simulink library "qrd_matrix_library"  (Simulink 8.7)
settings: Solver=ode45  StartTime=0.0  StopTime=10.0  RelTol=1e-3
values from neighbouring files (symbols this model uses):
  vectorization = 2    [qrd_test.m]
undefined symbols (not defined in the file or in its folder): AdvDSPBChannelOutDisplay, AdvDSPBDMemDisplay, Back_Substitution_instances, column_count, column_count_1, column_count_2, dpoly, dspba_ChannelInVis, dspba_ChannelOutVis, dspba_internal_get_channel_ports, evalAionMaskParam, latency, primtype, QRD_vectorization, recipsqrt, row, row_count, row_count_1, row_count_2, UseDontCare, value, x
libraries: DSPBAPrim x683, DSPBAControl x37, qrd_matrix_library x33, DSPBAVectorUtil x6, DSPBAVectorPrim x3
(part 6 of 8)

== system qrd_matrix_library/QR_decomposition/Data Mux ==
  Valid In : Inport
  Channel In : Inport  Port=2
  r2_k_k_valid_in : Inport  Port=3
  rn_k_j_valid_in : Inport  Port=4
  A_j_update_valid_in : Inport  Port=5
  Q_k_valid_in : Inport  Port=6
  Input_Memory_Read_Data : Inport  Port=7
  A_k_Memory_Read_Data : Inport  Port=8
  rn_k_j_over_r2_k_k_fifo_Data : Inport  Port=9
  inv_r_k_k_Data : Inport  Port=10
  Dot_Product_Acc_Init_In : Inport  Port=11
  r2_k_k_Acc_Valid_In : Inport  Port=12
  rn_k_j_Acc_Valid_In : Inport  Port=13
  A_j_Address_In : Inport  Port=14
  A_j_Update_last_Valid_In : Inport  Port=15
  Done_In : Inport  Port=16
  ChannelIn : DSPBAPrim/ChannelIn  primtype=channelin  nInputs=dspba_internal_get_channel_ports(gcb)  nOutputs=dspba_internal_get_channel_ports(gcb)  omode=Inherit via internal rule  otype=sfix(16)  scale=2^-15  rndmethod=Unbiased  factor=1  satmethod=Symmetric  shift_vec=[0 1 2 -1]  value=14  inPortNames=['v'; 'c'; '0'; '1'; '2'; '3'; '4'; '5'; '6'; '7'; '8'; '9'; 'A'; 'B'; 'D'; 'E'; 'F'; 'G'; 'H'; 'I'; 'J'; 'K'; 'L'; 'M'; 'N'; 'O'; 'P'; 'Q'; 'R'; 'S'; 'T'; 'U'; 'W'; 'X'; 'Y'; 'Z']  outPortNames=['v'; 'c'; '0'; '1'; '2'; '3'; '4'; '5'; '6'; '7'; '8'; '9'; 'A'; 'B'; 'D'; 'E'; 'F'; 'G'; 'H'; 'I'; 'J'; 'K'; 'L'; 'M'; 'N'; 'O'; 'P'; 'Q'; 'R'; 'S'; 'T'; 'U'; 'W'; 'X'; 'Y'; 'Z']  dspbaimage=dspba_prim.jpg  text=fprintf('In');  style=Optimised  dataSignals=14  foldingEnabled=off  channels=1  sampleRate=200  packetBeginPresent=off  packetBeginEnabled=off  visibilities=dspba_ChannelInVis(gcb)  latencyCorrection=0  version=20141013
  ChannelOut : DSPBAPrim/ChannelOut  primtype=channelout  nInputs=dspba_internal_get_channel_ports(gcb)  nOutputs=dspba_internal_get_channel_ports(gcb)  omode=Inherit via internal rule  otype=sfix(16)  scale=2^-15  rndmethod=Unbiased  factor=1  satmethod=Symmetric  shift_vec=[0 1 2 -1]  value=11  inPortNames=['v'; 'c'; '0'; '1'; '2'; '3'; '4'; '5'; '6'; '7'; '8'; '9'; 'A'; 'B'; 'D'; 'E'; 'F'; 'G'; 'H'; 'I'; 'J'; 'K'; 'L'; 'M'; 'N'; 'O'; 'P'; 'Q'; 'R'; 'S'; 'T'; 'U'; 'W'; 'X'; 'Y'; 'Z']  outPortNames=['v'; 'c'; '0'; '1'; '2'; '3'; '4'; '5'; '6'; '7'; '8'; '9'; 'A'; 'B'; 'D'; 'E'; 'F'; 'G'; 'H'; 'I'; 'J'; 'K'; 'L'; 'M'; 'N'; 'O'; 'P'; 'Q'; 'R'; 'S'; 'T'; 'U'; 'W'; 'X'; 'Y'; 'Z']  dspbaimage=dspba_prim.jpg  text=fprintf('Out%s', AdvDSPBChannelOutDisplay(latency));  style=Optimised  dataSignals=11  foldingEnabled=off  channels=1  sampleRate=200  packetBeginPresent=off  packetBeginEnabled=off  visibilities=dspba_ChannelOutVis(gcb)  latency=0  latencyCorrection=0  version=20141013
  ComplexConjugate : DSPBAPrim/ComplexConjugate  primtype=complexconjugate  nInputs=1  nOutputs=1  omode=Inherit via internal rule  otype=sfix(16)  scale=2^-15  rndmethod=Unbiased  factor=1  satmethod=Symmetric  shift_vec=[0 1 2 -1]  value=round([0:255]/17)  inPortNames=[' '; ' ';]  outPortNames=[' ']  dspbaimage=dspba_prim.jpg  text=fprintf('conj');  style=Optimised  visibilities=8  version=20090407
  ComplexConjugate1 : DSPBAPrim/ComplexConjugate  primtype=complexconjugate  nInputs=1  nOutputs=1  omode=Inherit via internal rule  otype=sfix(16)  scale=2^-15  rndmethod=Unbiased  factor=1  satmethod=Symmetric  shift_vec=[0 1 2 -1]  value=round([0:255]/17)  inPortNames=[' '; ' ';]  outPortNames=[' ']  dspbaimage=dspba_prim.jpg  text=fprintf('conj');  style=Optimised  visibilities=8  version=20090407
  Const11 : DSPBAPrim/Const  primtype=const  nInputs=0  nOutputs=1  omode=single  otype=uint(8)  scale=1  rndmethod=Unbiased  factor=1  satmethod=Symmetric  shift_vec=[0 1 2 -1]  value=0  inPortNames=['+'; '+';]  outPortNames=[' ']  dspbaimage=dspba_prim.jpg  text=fprintf('%s', num2str(value));  style=Optimised  visibilities=8 + 1024  floatPrecision=float32_m23  version=20120820
  Data1 Select : DSPBAPrim/Select  primtype=select  nInputs=str2num(get_param(gcb,'value'))*2+1  nOutputs=1  omode=Inherit via internal rule  otype=sfix(16)  scale=2^-15  rndmethod=Unbiased  factor=1  satmethod=Symmetric  shift_vec=[0 1 2 -1]  value=4  inPortNames=['d'; '0'; 'a'; '1'; 'b'; '2'; 'c'; '3'; 'd'; '4'; 'e'; '5'; 'f'; '6'; 'g'; '7'; 'h'; '8'; 'i'; '9'; 'j']  outPortNames=[' ']  dspbaimage=dspba_prim.jpg  text=fprintf('%s', primtype);  style=Optimised  visibilities=8 + 1024  version=20090407
  Data2 Select : DSPBAPrim/Select  primtype=select  nInputs=str2num(get_param(gcb,'value'))*2+1  nOutputs=1  omode=Inherit via internal rule  otype=sfix(16)  scale=2^-15  rndmethod=Unbiased  factor=1  satmethod=Symmetric  shift_vec=[0 1 2 -1]  value=4  inPortNames=['d'; '0'; 'a'; '1'; 'b'; '2'; 'c'; '3'; 'd'; '4'; 'e'; '5'; 'f'; '6'; 'g'; '7'; 'h'; '8'; 'i'; '9'; 'j']  outPortNames=[' ']  dspbaimage=dspba_prim.jpg  text=fprintf('%s', primtype);  style=Optimised  visibilities=8 + 1024  version=20090407
  ExpandScalar : DSPBAVectorUtil/ExpandScalar  vecWidth=vectorization
  Real-Imag to Complex : RealImagToComplex
  SynthesisInfo : DSPBAPrim/SynthesisInfo  primtype=synthinfo  nInputs=0  nOutputs=0  omode=Inherit via internal rule  otype=sfix(16)  scale=2^-15  rndmethod=Truncate  factor=1  satmethod=Symmetric  shift_vec=[0 1 2 -1]  value=99  inPortNames=[' '; ' ';]  outPortNames=[' ']  dspbaimage=dspba_prim_ctrl.jpg  text=fprintf('Style=%s', style);  style=Scheduled  visibilities=2^17+2^18+2^19+2^20  constraintInUse=off  constraintRelation=>  constraintLimit=2  bitAccurate=off  version=20150220
  Valid Out : Outport
  Data Out 1 : Outport  Port=2
  Data Out 2 : Outport  Port=3
  Dot_Product_Acc_Init_Out : Outport  Port=4
  r2_k_k_Acc_Valid_Out : Outport  Port=5
  rn_k_j_Acc_Valid_Out : Outport  Port=6
  A_j_update_valid_Out : Outport  Port=7
  Q_k_valid_Out : Outport  Port=8
  Input_Memory_Read_Data_Out : Outport  Port=9
  A_j_Address_Out : Outport  Port=10
  A_j_Update_last_Valid_Out : Outport  Port=11
  Done_Out : Outport  Port=12
  wires:
  ChannelIn/7 -> ComplexConjugate/1, ChannelOut/10, Data2 Select/5, Data2 Select/3
  ChannelIn/1 -> ChannelOut/1
  Valid In/1 -> ChannelIn/1
  ChannelIn/11 -> ChannelOut/5
  Q_k_valid_in/1 -> ChannelIn/6
  Input_Memory_Read_Data/1 -> ChannelIn/7
  rn_k_j_over_r2_k_k_fifo_Data/1 -> ChannelIn/9
  ComplexConjugate1/1 -> Data1 Select/5
  ComplexConjugate/1 -> Data1 Select/3
  ChannelIn/8 -> ComplexConjugate1/1, Data1 Select/9, Data2 Select/7
  Data2 Select/1 -> ChannelOut/4
  Dot_Product_Acc_Init_In/1 -> ChannelIn/11
  inv_r_k_k_Data/1 -> ChannelIn/10
  ChannelIn/5 -> ChannelOut/8, Data2 Select/6, Data1 Select/6
  ChannelOut/6 -> r2_k_k_Acc_Valid_Out/1
  Data1 Select/1 -> ChannelOut/3
  ChannelIn/12 -> ChannelOut/6
  ChannelOut/3 -> Data Out 1/1
  ChannelOut/5 -> Dot_Product_Acc_Init_Out/1
  ChannelIn/3 -> Data1 Select/2, Data2 Select/2
  Channel In/1 -> ChannelIn/2
  ChannelOut/4 -> Data Out 2/1
  ChannelIn/13 -> ChannelOut/7
  ChannelIn/4 -> Data2 Select/4, Data1 Select/4
  ChannelIn/2 -> ChannelOut/2
  ChannelOut/1 -> Valid Out/1
  ChannelIn/9 -> Data1 Select/7
  ChannelOut/7 -> rn_k_j_Acc_Valid_Out/1
  A_k_Memory_Read_Data/1 -> ChannelIn/8
  r2_k_k_valid_in/1 -> ChannelIn/3
  rn_k_j_valid_in/1 -> ChannelIn/4
  A_j_update_valid_in/1 -> ChannelIn/5
  r2_k_k_Acc_Valid_In/1 -> ChannelIn/12
  ChannelIn/14 -> ChannelOut/11
  ChannelOut/9 -> Q_k_valid_Out/1
  rn_k_j_Acc_Valid_In/1 -> ChannelIn/13
  ChannelOut/10 -> Input_Memory_Read_Data_Out/1
  ChannelIn/15 -> ChannelOut/12
  ChannelOut/11 -> A_j_Address_Out/1
  ChannelOut/8 -> A_j_update_valid_Out/1
  A_j_Address_In/1 -> ChannelIn/14
  A_j_Update_last_Valid_In/1 -> ChannelIn/15
  ChannelIn/10 -> Data2 Select/9
  ChannelIn/6 -> ChannelOut/9, Data2 Select/8, Data1 Select/8
  ChannelOut/12 -> A_j_Update_last_Valid_Out/1
  Done_In/1 -> ChannelIn/16
  ChannelOut/13 -> Done_Out/1
  ChannelIn/16 -> ChannelOut/13
  Const11/1 -> Real-Imag to Complex/1, Real-Imag to Complex/2
  Real-Imag to Complex/1 -> ExpandScalar/1
  ExpandScalar/1 -> Data1 Select/1, Data2 Select/1

== system qrd_matrix_library/QR_decomposition/Dot Product ==
  Valid_In : Inport
  Channel_In : Inport  Port=2
  Data_In1 : Inport  Port=3
  Data_In2 : Inport  Port=4
  Acc_Init : Inport  Port=5
  r2_k_k_valid_in : Inport  Port=6
  rn_k_j_valid_in : Inport  Port=7
  A_j_update_valid_in : Inport  Port=8
  Q_k_valid_in : Inport  Port=9
  A_j_Read_Data_In : Inport  Port=10
  A_j_Address_In : Inport  Port=11
  A_j_Update_last_Valid_In : Inport  Port=12
  Done_In : Inport  Port=13
  Acc : DSPBAPrim/Acc  primtype=acc  nInputs=2  nOutputs=4  omode=Inherit via internal rule  otype=sfix(16)  scale=2^-15  rndmethod=Unbiased  factor=1  satmethod=Symmetric  shift_vec=[0 1 2 -1]  value=[-26 20 12]  inPortNames=['x';'n']  outPortNames=['r ';'xO';'xU';'aO';]  dspbaimage=dspba_prim_float.jpg  text=fprintf('acc(x)');  style=Optimised  visibilities=1024  version=20090407
  And : DSPBAPrim/And  Commented=on  primtype=and  nInputs=2  nOutputs=1  omode=Inherit via internal rule  otype=sfix(16)  scale=2^-15  rndmethod=Unbiased  factor=1  satmethod=Symmetric  shift_vec=[0 1 2 -1]  value=0  inPortNames=[' '; ' '; ' '; ' '; ' '; ' '; ' '; ' '; ' '; ' '; ' '; ' '; ' '; ' '; ' '; ' '; ]  outPortNames=[' ']  dspbaimage=dspba_prim.jpg  text=fprintf('&');  style=Optimised  visibilities=8+2  version=20090407
  ChannelIn : DSPBAPrim/ChannelIn  primtype=channelin  nInputs=dspba_internal_get_channel_ports(gcb)  nOutputs=dspba_internal_get_channel_ports(gcb)  omode=Inherit via internal rule  otype=sfix(16)  scale=2^-15  rndmethod=Unbiased  factor=1  satmethod=Symmetric  shift_vec=[0 1 2 -1]  value=11  inPortNames=['v'; 'c'; '0'; '1'; '2'; '3'; '4'; '5'; '6'; '7'; '8'; '9'; 'A'; 'B'; 'D'; 'E'; 'F'; 'G'; 'H'; 'I'; 'J'; 'K'; 'L'; 'M'; 'N'; 'O'; 'P'; 'Q'; 'R'; 'S'; 'T'; 'U'; 'W'; 'X'; 'Y'; 'Z']  outPortNames=['v'; 'c'; '0'; '1'; '2'; '3'; '4'; '5'; '6'; '7'; '8'; '9'; 'A'; 'B'; 'D'; 'E'; 'F'; 'G'; 'H'; 'I'; 'J'; 'K'; 'L'; 'M'; 'N'; 'O'; 'P'; 'Q'; 'R'; 'S'; 'T'; 'U'; 'W'; 'X'; 'Y'; 'Z']  dspbaimage=dspba_prim.jpg  text=fprintf('In');  style=Optimised  dataSignals=11  foldingEnabled=off  channels=1  sampleRate=200  packetBeginPresent=off  packetBeginEnabled=off  visibilities=dspba_ChannelInVis(gcb)  latencyCorrection=0  version=20141013
  Complex to Real-Imag : ComplexToRealImag
  Const7 : DSPBAPrim/Const  primtype=const  nInputs=0  nOutputs=1  omode=Specify via dialog  otype=uint(8)  scale=1  rndmethod=Unbiased  factor=1  satmethod=Symmetric  shift_vec=[0 1 2 -1]  value=0  inPortNames=['+'; '+';]  outPortNames=[' ']  dspbaimage=dspba_prim.jpg  text=fprintf('%s', num2str(value));  style=Optimised  visibilities=8 + 1024  floatPrecision=float32_m23  version=20120820
  Demux : Demux  Outputs=2
  Dot Product ChannelOut : DSPBAPrim/ChannelOut  primtype=channelout  nInputs=dspba_internal_get_channel_ports(gcb)  nOutputs=dspba_internal_get_channel_ports(gcb)  omode=Inherit via internal rule  otype=sfix(16)  scale=2^-15  rndmethod=Unbiased  factor=1  satmethod=Symmetric  shift_vec=[0 1 2 -1]  value=3  inPortNames=['v'; 'c'; '0'; '1'; '2'; '3'; '4'; '5'; '6'; '7'; '8'; '9'; 'A'; 'B'; 'D'; 'E'; 'F'; 'G'; 'H'; 'I'; 'J'; 'K'; 'L'; 'M'; 'N'; 'O'; 'P'; 'Q'; 'R'; 'S'; 'T'; 'U'; 'W'; 'X'; 'Y'; 'Z']  outPortNames=['v'; 'c'; '0'; '1'; '2'; '3'; '4'; '5'; '6'; '7'; '8'; '9'; 'A'; 'B'; 'D'; 'E'; 'F'; 'G'; 'H'; 'I'; 'J'; 'K'; 'L'; 'M'; 'N'; 'O'; 'P'; 'Q'; 'R'; 'S'; 'T'; 'U'; 'W'; 'X'; 'Y'; 'Z']  dspbaimage=dspba_prim.jpg  text=fprintf('Out%s', AdvDSPBChannelOutDisplay(latency));  style=Optimised  dataSignals=3  foldingEnabled=off  channels=1  sampleRate=200  packetBeginPresent=off  packetBeginEnabled=off  visibilities=dspba_ChannelOutVis(gcb)  latency=0  latencyCorrection=0  version=20141013
  Mult : DSPBAPrim/Mult  primtype=mult  nInputs=2  nOutputs=1  omode=Inherit via internal rule  otype=sfix(16)  scale=2^-15  rndmethod=Unbiased  factor=1  satmethod=Symmetric  shift_vec=[0 1 2 -1]  value=0  inPortNames=[' '; ' ';]  outPortNames=[' ']  dspbaimage=dspba_prim.jpg  text=fprintf('X');  style=Optimised  visibilities=8+2^18+2^19  floatPrecision=float32_m23  floatRounding=correct  advOptions=[]  version=20130115
  Mult ChannelOut : DSPBAPrim/ChannelOut  primtype=channelout  nInputs=dspba_internal_get_channel_ports(gcb)  nOutputs=dspba_internal_get_channel_ports(gcb)  omode=Inherit via internal rule  otype=sfix(16)  scale=2^-15  rndmethod=Unbiased  factor=1  satmethod=Symmetric  shift_vec=[0 1 2 -1]  value=7  inPortNames=['v'; 'c'; '0'; '1'; '2'; '3'; '4'; '5'; '6'; '7'; '8'; '9'; 'A'; 'B'; 'D'; 'E'; 'F'; 'G'; 'H'; 'I'; 'J'; 'K'; 'L'; 'M'; 'N'; 'O'; 'P'; 'Q'; 'R'; 'S'; 'T'; 'U'; 'W'; 'X'; 'Y'; 'Z']  outPortNames=['v'; 'c'; '0'; '1'; '2'; '3'; '4'; '5'; '6'; '7'; '8'; '9'; 'A'; 'B'; 'D'; 'E'; 'F'; 'G'; 'H'; 'I'; 'J'; 'K'; 'L'; 'M'; 'N'; 'O'; 'P'; 'Q'; 'R'; 'S'; 'T'; 'U'; 'W'; 'X'; 'Y'; 'Z']  dspbaimage=dspba_prim.jpg  text=fprintf('Out%s', AdvDSPBChannelOutDisplay(latency));  style=Optimised  dataSignals=7  foldingEnabled=off  channels=1  sampleRate=200  packetBeginPresent=off  packetBeginEnabled=off  visibilities=dspba_ChannelOutVis(gcb)  latency=0  latencyCorrection=0  version=20141013
  MultAcc : DSPBAPrim/MultAcc  Commented=on  primtype=multaccfunc  nInputs=3  nOutputs=1  omode=Inherit via internal rule  otype=sfix(16)  scale=2^-15  rndmethod=Unbiased  factor=1  satmethod=Symmetric  shift_vec=[0 1 2 -1]  value=0  inPortNames="[ 'acc'; 'x  '; 'y  ']"  outPortNames=[]  dspbaimage=dspba_prim_float.jpg  text=disp('multAcc');  style=Optimised  visibilities=8+2^17  functionExpr=fpAcc  advOptions=[]  version=20121130
  Mux : Mux  Inputs=2
  Not : DSPBAPrim/Not  Commented=on  primtype=not  nInputs=1  nOutputs=1  omode=Inherit via internal rule  otype=sfix(16)  scale=2^-15  rndmethod=Unbiased  factor=1  satmethod=Symmetric  shift_vec=[0 1 2 -1]  value=0  inPortNames=[' '; ' ';]  outPortNames=[' ']  dspbaimage=dspba_prim.jpg  text=fprintf('~');  style=Optimised  visibilities=8  version=20090407
  Or : DSPBAPrim/Or  primtype=or  nInputs=2  nOutputs=1  omode=Inherit via internal rule  otype=sfix(16)  scale=2^-15  rndmethod=Unbiased  factor=1  satmethod=Symmetric  shift_vec=[0 1 2 -1]  value=0  inPortNames=[' '; ' '; ' '; ' '; ' '; ' '; ' '; ' '; ' '; ' '; ' '; ' '; ' '; ' '; ' '; ' '; ]  outPortNames=[' ']  dspbaimage=dspba_prim.jpg  text=fprintf('|');  style=Optimised  visibilities=8+2  version=20090407
  Or1 : DSPBAPrim/Or  primtype=or  nInputs=2  nOutputs=1  omode=Inherit via internal rule  otype=sfix(16)  scale=2^-15  rndmethod=Unbiased  factor=1  satmethod=Symmetric  shift_vec=[0 1 2 -1]  value=0  inPortNames=[' '; ' '; ' '; ' '; ' '; ' '; ' '; ' '; ' '; ' '; ' '; ' '; ' '; ' '; ' '; ' '; ]  outPortNames=[' ']  dspbaimage=dspba_prim.jpg  text=fprintf('|');  style=Optimised  visibilities=8+2  version=20090407
  Real-Imag to Complex : RealImagToComplex
  ReinterpretCast : DSPBAPrim/ReinterpretCast  primtype=reinterpret  nInputs=1  nOutputs=1  omode=single  otype=sfix(16)  scale=2^-15  rndmethod=Unbiased  factor=1  satmethod=Symmetric  shift_vec=[0 1 2 -1]  value=0  inPortNames=[' '; ' ';]  outPortNames=[' ']  dspbaimage=dspba_prim.jpg  text=fprintf('Reinterp\nCast', value);  style=Optimised  visibilities=8  floatPrecision=float32_m23  version=20120601
  SumOfElements : DSPBAVectorPrim/SumOfElements  primtype=sumofelements  nInputs=1  nOutputs=1  omode=Inherit via internal rule with word growth  otype=sfix(16)  scale=2^-15  rndmethod=Unbiased  factor=1  satmethod=Symmetric  shift_vec=[0 1 2 -1]  value=1  inPortNames=[' '; ' ';]  outPortNames=[' ']  dspbaimage=dspba_prim.jpg  text=fprintf('+');  style=Optimised  visibilities=8+2^17+2^18+2^19  genFPC=off  floatRounding=correct  advOptions=[]  version=20130821
  SynthesisInfo : DSPBAPrim/SynthesisInfo  primtype=synthinfo  nInputs=0  nOutputs=0  omode=Inherit via internal rule  otype=sfix(16)  scale=2^-15  rndmethod=Truncate  factor=1  satmethod=Symmetric  shift_vec=[0 1 2 -1]  value=99  inPortNames=[' '; ' ';]  outPortNames=[' ']  dspbaimage=dspba_prim_ctrl.jpg  text=fprintf('Style=%s', style);  style=Scheduled  visibilities=2^17+2^18+2^19+2^20  constraintInUse=off  constraintRelation=>  constraintLimit=2  bitAccurate=off  version=20150220
  latch_0L : DSPBAControl/latch_0L
  Dot Product Valid_Out : Outport
  Dot Product Data_Out : Outport  Port=2
  r2_k_k_valid_out : Outport  Port=3
  rn_k_j_valid_out : Outport  Port=4
  Mult Valid_out : Outport  Port=5
  Mult Data_out : Outport  Port=6
  A_j_update_valid_Out : Outport  Port=7
  Q_k_valid_Out : Outport  Port=8
  A_j_Read_Data_Out : Outport  Port=9
  A_j_Address_Out : Outport  Port=10
  A_j_Update_last_Valid_Out : Outport  Port=11
  Done_Out : Outport  Port=12
  wires:
  ChannelIn/6 -> Or1/1, Dot Product ChannelOut/4
  Data_In1/1 -> ChannelIn/3
  Valid_In/1 -> ChannelIn/1
  ChannelIn/5 -> Acc/2
  Demux/2 -> Real-Imag to Complex/2
  Mux/1 -> Acc/1
  Acc/1 -> Demux/1
  ChannelIn/4 -> Mult/2
  Channel_In/1 -> ChannelIn/2
  Complex to Real-Imag/2 -> Mux/2
  Mult/1 -> Mult ChannelOut/3, SumOfElements/1
  SumOfElements/1 -> Complex to Real-Imag/1
  Real-Imag to Complex/1 -> ReinterpretCast/1
  Acc_Init/1 -> ChannelIn/5
  Complex to Real-Imag/1 -> Mux/1
  r2_k_k_valid_in/1 -> ChannelIn/6
  Demux/1 -> Real-Imag to Complex/1
  ChannelIn/3 -> Mult/1
  Dot Product ChannelOut/1 -> Dot Product Valid_Out/1
  Dot Product ChannelOut/3 -> Dot Product Data_Out/1
  Data_In2/1 -> ChannelIn/4
  rn_k_j_valid_in/1 -> ChannelIn/7
  Q_k_valid_in/1 -> ChannelIn/9
  ChannelIn/2 -> Dot Product ChannelOut/2
  ChannelIn/7 -> Or1/2, Dot Product ChannelOut/5
  ChannelIn/10 -> Mult ChannelOut/6
  Dot Product ChannelOut/4 -> r2_k_k_valid_out/1
  Dot Product ChannelOut/5 -> rn_k_j_valid_out/1
  Mult ChannelOut/4 -> A_j_update_valid_Out/1
  Const7/1 -> Mult ChannelOut/2
  ChannelIn/1 -> Dot Product ChannelOut/1
  Mult ChannelOut/1 -> Mult Valid_out/1
  Mult ChannelOut/3 -> Mult Data_out/1
  A_j_Read_Data_In/1 -> ChannelIn/10
  Mult ChannelOut/5 -> Q_k_valid_Out/1
  ChannelIn/11 -> Mult ChannelOut/7
  A_j_Address_In/1 -> ChannelIn/11
  Mult ChannelOut/6 -> A_j_Read_Data_Out/1
  ChannelIn/12 -> Mult ChannelOut/8
  ChannelIn/8 -> Or/1, Mult ChannelOut/4
  A_j_update_valid_in/1 -> ChannelIn/8
  A_j_Update_last_Valid_In/1 -> ChannelIn/12
  Mult ChannelOut/8 -> A_j_Update_last_Valid_Out/1
  Mult ChannelOut/7 -> A_j_Address_Out/1
  ChannelIn/9 -> Mult ChannelOut/5, Or/2
  Or/1 -> Mult ChannelOut/1
  Done_In/1 -> ChannelIn/13
  Mult ChannelOut/9 -> Done_Out/1
  ChannelIn/13 -> Mult ChannelOut/9
  And/1 -> ?
  Not/1 -> And/2
  ReinterpretCast/1 -> latch_0L/2
  latch_0L/1 -> Dot Product ChannelOut/3
  Or1/1 -> latch_0L/1

== system qrd_matrix_library/QR_decomposition/Input Memory Controller ==
  External Write : Inport
  External Write Address : Inport  Port=2
  External Write Data : Inport  Port=3
  Input_A_k_Read_Valid : Inport  Port=4
  Input_A_k_Read_Address : Inport  Port=5
  Input_A_j_Read_Valid1 : Inport  Port=6
  Input_A_j_Read_Address1 : Inport  Port=7
  Input_A_j_Read_Valid2 : Inport  Port=8
  Input_A_j_Read_Address2 : Inport  Port=9
  Feedback Write : Inport  Port=10
  Feedback Address : Inport  Port=11
  Feedback Data : Inport  Port=12
  Const3 : DSPBAPrim/Const  primtype=const  nInputs=0  nOutputs=1  omode=Inherit via internal rule  otype=sfix(16)  scale=2^-15  rndmethod=Unbiased  factor=1  satmethod=Symmetric  shift_vec=[0 1 2 -1]  value=0  inPortNames=['+'; '+';]  outPortNames=[' ']  dspbaimage=dspba_prim.jpg  text=fprintf('%s', num2str(value));  style=Optimised  visibilities=8 + 1024  floatPrecision=float32_m23  version=20120820
  Input Memory Read 2 Address Select : DSPBAPrim/Select  primtype=select  nInputs=str2num(get_param(gcb,'value'))*2+1  nOutputs=1  omode=Inherit via internal rule  otype=sfix(16)  scale=2^-15  rndmethod=Unbiased  factor=1  satmethod=Symmetric  shift_vec=[0 1 2 -1]  value=3  inPortNames=['d'; '0'; 'a'; '1'; 'b'; '2'; 'c'; '3'; 'd'; '4'; 'e'; '5'; 'f'; '6'; 'g'; '7'; 'h'; '8'; 'i'; '9'; 'j']  outPortNames=[' ']  dspbaimage=dspba_prim.jpg  text=fprintf('%s', primtype);  style=Optimised  visibilities=8 + 1024  version=20090407
  Input Memory Write Address Select : DSPBAPrim/Select  primtype=select  nInputs=str2num(get_param(gcb,'value'))*2+1  nOutputs=1  omode=Inherit via internal rule  otype=sfix(16)  scale=2^-15  rndmethod=Unbiased  factor=1  satmethod=Symmetric  shift_vec=[0 1 2 -1]  value=2  inPortNames=['d'; '0'; 'a'; '1'; 'b'; '2'; 'c'; '3'; 'd'; '4'; 'e'; '5'; 'f'; '6'; 'g'; '7'; 'h'; '8'; 'i'; '9'; 'j']  outPortNames=[' ']  dspbaimage=dspba_prim.jpg  text=fprintf('%s', primtype);  style=Optimised  visibilities=8 + 1024  version=20090407
  Input Memory Write Data Select : DSPBAPrim/Select  primtype=select  nInputs=str2num(get_param(gcb,'value'))*2+1  nOutputs=1  omode=Inherit via internal rule  otype=sfix(16)  scale=2^-15  rndmethod=Unbiased  factor=1  satmethod=Symmetric  shift_vec=[0 1 2 -1]  value=2  inPortNames=['d'; '0'; 'a'; '1'; 'b'; '2'; 'c'; '3'; 'd'; '4'; 'e'; '5'; 'f'; '6'; 'g'; '7'; 'h'; '8'; 'i'; '9'; 'j']  outPortNames=[' ']  dspbaimage=dspba_prim.jpg  text=fprintf('%s', primtype);  style=Optimised  visibilities=8 + 1024  version=20090407
  Input RAM : DSPBAPrim/DualMem  primtype=dualmem  nInputs=4  nOutputs=2  omode=single  otype=sfix(16)  scale=2^-15  rndmethod=Unbiased  factor=1  satmethod=Symmetric  shift_vec=[0 1 2 -1]  value=complex(zeros((size*size)/vectorization,vectorization),zeros((size*size)/vectorization,vectorization))  inPortNames=['d1'; 'a1'; 'w1'; 'a2']  outPortNames=['q1'; 'q2']  dspbaimage=dspba_prim.jpg  text=fprintf('dmem%s',AdvDSPBDMemDisplay(UseDontCare));  style=Optimised  visibilities=8 + 1024 + 2^17 + 2^18  UseDontCare=off  TwinWritePorts=off  version=20141001
  Select Delay : DSPBAPrim/SampleDelay  primtype=sampdelay  nInputs=1  nOutputs=1  omode=Inherit via internal rule  otype=sfix(16)  scale=2^-15  rndmethod=Unbiased  factor=1  satmethod=Symmetric  shift_vec=[0 1 2 -1]  value=1  inPortNames=[' '; ' ';]  outPortNames=[' ']  dspbaimage=dspba_prim.jpg  text=dpoly(1, eye(1,value+1), 'z')  style=Optimised  visibilities=8 + 1024 + 2^17 + 2^18  flexible=off  slackgroup=0  augmented=0  version=20090407  advOptions=[]
  Write_Valid_Or : DSPBAPrim/Or  primtype=or  nInputs=2  nOutputs=1  omode=Inherit via internal rule  otype=sfix(16)  scale=2^-15  rndmethod=Unbiased  factor=1  satmethod=Symmetric  shift_vec=[0 1 2 -1]  value=0  inPortNames=[' '; ' '; ' '; ' '; ' '; ' '; ' '; ' '; ' '; ' '; ' '; ' '; ' '; ' '; ' '; ' '; ]  outPortNames=[' ']  dspbaimage=dspba_prim.jpg  text=fprintf('|');  style=Optimised  visibilities=8+2  version=20090407
  Read Data : Outport
  wires:
  Input_A_k_Read_Address/1 -> Input Memory Read 2 Address Select/3
  Input RAM/2 -> Read Data/1
  Input_A_k_Read_Valid/1 -> Input Memory Read 2 Address Select/2
  Input_A_j_Read_Valid1/1 -> Input Memory Read 2 Address Select/4
  Input_A_j_Read_Address1/1 -> Input Memory Read 2 Address Select/5
  Input Memory Read 2 Address Select/1 -> Input RAM/4
  Const3/1 -> Input Memory Read 2 Address Select/1
  Input_A_j_Read_Valid2/1 -> Input Memory Read 2 Address Select/6
  Input_A_j_Read_Address2/1 -> Input Memory Read 2 Address Select/7
  External Write Address/1 -> Input Memory Write Address Select/1, Input Memory Write Address Select/3
  External Write/1 -> Input Memory Write Data Select/2, Write_Valid_Or/1, Input Memory Write Address Select/2
  External Write Data/1 -> Input Memory Write Data Select/1, Input Memory Write Data Select/3
  Input Memory Write Address Select/1 -> Input RAM/2
  Input Memory Write Data Select/1 -> Input RAM/1
  Write_Valid_Or/1 -> Select Delay/1
  Select Delay/1 -> Input RAM/3
  Feedback Write/1 -> Write_Valid_Or/2, Input Memory Write Data Select/4, Input Memory Write Address Select/4
  Feedback Address/1 -> Input Memory Write Address Select/5
  Feedback Data/1 -> Input Memory Write Data Select/5

== system qrd_matrix_library/QR_decomposition/Inv SQRT ==
  Valid In : Inport
  Channel In : Inport  Port=2
  r2_k_k : Inport  Port=3
  ChannelIn : DSPBAPrim/ChannelIn  primtype=channelin  nInputs=dspba_internal_get_channel_ports(gcb)  nOutputs=dspba_internal_get_channel_ports(gcb)  omode=Inherit via internal rule  otype=sfix(16)  scale=2^-15  rndmethod=Unbiased  factor=1  satmethod=Symmetric  shift_vec=[0 1 2 -1]  value=1  inPortNames=['v'; 'c'; '0'; '1'; '2'; '3'; '4'; '5'; '6'; '7'; '8'; '9'; 'A'; 'B'; 'D'; 'E'; 'F'; 'G'; 'H'; 'I'; 'J'; 'K'; 'L'; 'M'; 'N'; 'O'; 'P'; 'Q'; 'R'; 'S'; 'T'; 'U'; 'W'; 'X'; 'Y'; 'Z']  outPortNames=['v'; 'c'; '0'; '1'; '2'; '3'; '4'; '5'; '6'; '7'; '8'; '9'; 'A'; 'B'; 'D'; 'E'; 'F'; 'G'; 'H'; 'I'; 'J'; 'K'; 'L'; 'M'; 'N'; 'O'; 'P'; 'Q'; 'R'; 'S'; 'T'; 'U'; 'W'; 'X'; 'Y'; 'Z']  dspbaimage=dspba_prim.jpg  text=fprintf('In');  style=Optimised  dataSignals=1  foldingEnabled=off  channels=1  sampleRate=200  packetBeginPresent=off  packetBeginEnabled=off  visibilities=dspba_ChannelInVis(gcb)  latencyCorrection=0  version=20141013
  Complex to Real-Imag : ComplexToRealImag
  Mult : DSPBAPrim/Mult  primtype=mult  nInputs=2  nOutputs=1  omode=Inherit via internal rule  otype=sfix(16)  scale=2^-15  rndmethod=Unbiased  factor=1  satmethod=Symmetric  shift_vec=[0 1 2 -1]  value=0  inPortNames=[' '; ' ';]  outPortNames=[' ']  dspbaimage=dspba_prim.jpg  text=fprintf('X');  style=Optimised  visibilities=8+2^18+2^19  floatPrecision=float32_m23  floatRounding=correct  advOptions=[]  version=20130115
  RecipSqRt : DSPBAPrim/Sqrt  primtype=sqrtfunc  nInputs=1  nOutputs=1  omode=Inherit via internal rule  otype=sfix(16)  scale=2^-15  rndmethod=Unbiased  factor=1  satmethod=Symmetric  shift_vec=[0 1 2 -1]  value=round([0:255]/17)  inPortNames=[' '; ' ';]  outPortNames=[' ']  dspbaimage=dspba_prim_float.jpg  text=fprintf('sqrt(x)');  style=Optimised  visibilities=2^17  functionExpr=recipsqrt(x)  floatRounding=correct  advOptions=[]  version=20120730
  SynthesisInfo : DSPBAPrim/SynthesisInfo  primtype=synthinfo  nInputs=0  nOutputs=0  omode=Inherit via internal rule  otype=sfix(16)  scale=2^-15  rndmethod=Truncate  factor=1  satmethod=Symmetric  shift_vec=[0 1 2 -1]  value=99  inPortNames=[' '; ' ';]  outPortNames=[' ']  dspbaimage=dspba_prim_ctrl.jpg  text=fprintf('Style=%s', style);  style=Scheduled  visibilities=2^17+2^18+2^19+2^20  constraintInUse=off  constraintRelation=>  constraintLimit=2  bitAccurate=off  version=20150220
  Terminator : Terminator
  inv_r2_k_k ChannelOut : DSPBAPrim/ChannelOut  primtype=channelout  nInputs=dspba_internal_get_channel_ports(gcb)  nOutputs=dspba_internal_get_channel_ports(gcb)  omode=Inherit via internal rule  otype=sfix(16)  scale=2^-15  rndmethod=Unbiased  factor=1  satmethod=Symmetric  shift_vec=[0 1 2 -1]  value=1  inPortNames=['v'; 'c'; '0'; '1'; '2'; '3'; '4'; '5'; '6'; '7'; '8'; '9'; 'A'; 'B'; 'D'; 'E'; 'F'; 'G'; 'H'; 'I'; 'J'; 'K'; 'L'; 'M'; 'N'; 'O'; 'P'; 'Q'; 'R'; 'S'; 'T'; 'U'; 'W'; 'X'; 'Y'; 'Z']  outPortNames=['v'; 'c'; '0'; '1'; '2'; '3'; '4'; '5'; '6'; '7'; '8'; '9'; 'A'; 'B'; 'D'; 'E'; 'F'; 'G'; 'H'; 'I'; 'J'; 'K'; 'L'; 'M'; 'N'; 'O'; 'P'; 'Q'; 'R'; 'S'; 'T'; 'U'; 'W'; 'X'; 'Y'; 'Z']  dspbaimage=dspba_prim.jpg  text=fprintf('Out%s', AdvDSPBChannelOutDisplay(latency));  style=Optimised  dataSignals=1  foldingEnabled=off  channels=1  sampleRate=200  packetBeginPresent=off  packetBeginEnabled=off  visibilities=dspba_ChannelOutVis(gcb)  latency=0  latencyCorrection=0  version=20141013
  inv_r2_k_k_latch_0L : DSPBAControl/latch_0L
  inv_r_k_k ChannelOut : DSPBAPrim/ChannelOut  primtype=channelout  nInputs=dspba_internal_get_channel_ports(gcb)  nOutputs=dspba_internal_get_channel_ports(gcb)  omode=Inherit via internal rule  otype=sfix(16)  scale=2^-15  rndmethod=Unbiased  factor=1  satmethod=Symmetric  shift_vec=[0 1 2 -1]  value=1  inPortNames=['v'; 'c'; '0'; '1'; '2'; '3'; '4'; '5'; '6'; '7'; '8'; '9'; 'A'; 'B'; 'D'; 'E'; 'F'; 'G'; 'H'; 'I'; 'J'; 'K'; 'L'; 'M'; 'N'; 'O'; 'P'; 'Q'; 'R'; 'S'; 'T'; 'U'; 'W'; 'X'; 'Y'; 'Z']  outPortNames=['v'; 'c'; '0'; '1'; '2'; '3'; '4'; '5'; '6'; '7'; '8'; '9'; 'A'; 'B'; 'D'; 'E'; 'F'; 'G'; 'H'; 'I'; 'J'; 'K'; 'L'; 'M'; 'N'; 'O'; 'P'; 'Q'; 'R'; 'S'; 'T'; 'U'; 'W'; 'X'; 'Y'; 'Z']  dspbaimage=dspba_prim.jpg  text=fprintf('Out%s', AdvDSPBChannelOutDisplay(latency));  style=Optimised  dataSignals=1  foldingEnabled=off  channels=1  sampleRate=200  packetBeginPresent=off  packetBeginEnabled=off  visibilities=dspba_ChannelOutVis(gcb)  latency=0  latencyCorrection=0  version=20141013
  inv_r_k_k_latch_0L : DSPBAControl/latch_0L
  inv_r_k_k_valid_out : Outport
  inv_r_k_k : Outport  Port=2
  inv_r2_k_k_valid_out : Outport  Port=3
  inv_r2_k_k : Outport  Port=4
  wires:
  Valid In/1 -> ChannelIn/1
  Channel In/1 -> ChannelIn/2
  r2_k_k/1 -> ChannelIn/3
  ChannelIn/3 -> Complex to Real-Imag/1
  RecipSqRt/1 -> Mult/2, Mult/1, inv_r_k_k_latch_0L/2
  ChannelIn/1 -> inv_r_k_k ChannelOut/1, inv_r_k_k_latch_0L/1, inv_r2_k_k_latch_0L/1, inv_r2_k_k ChannelOut/1
  inv_r_k_k ChannelOut/3 -> inv_r_k_k/1
  inv_r_k_k ChannelOut/1 -> inv_r_k_k_valid_out/1
  Mult/1 -> inv_r2_k_k_latch_0L/2
  ChannelIn/2 -> inv_r2_k_k ChannelOut/2, inv_r_k_k ChannelOut/2
  inv_r2_k_k ChannelOut/1 -> inv_r2_k_k_valid_out/1
  inv_r2_k_k ChannelOut/3 -> inv_r2_k_k/1
  Complex to Real-Imag/1 -> RecipSqRt/1
  inv_r_k_k_latch_0L/1 -> inv_r_k_k ChannelOut/3
  inv_r2_k_k_latch_0L/1 -> inv_r2_k_k ChannelOut/3
  Complex to Real-Imag/2 -> Terminator/1

== system qrd_matrix_library/QR_decomposition/Inv_Rk Output Memory Controller ==
  Write Enable : Inport
  Write Data : Inport  Port=2
  Wr_Addr_Clr : Inport  Port=3
  Done : Inport  Port=4
  Source Ready : Inport  Port=5
  Size : Inport  Port=6
  And : DSPBAPrim/And  primtype=and  nInputs=2  nOutputs=1  omode=Inherit via internal rule  otype=sfix(16)  scale=2^-15  rndmethod=Unbiased  factor=1  satmethod=Symmetric  shift_vec=[0 1 2 -1]  value=0  inPortNames=[' '; ' '; ' '; ' '; ' '; ' '; ' '; ' '; ' '; ' '; ' '; ' '; ' '; ' '; ' '; ' '; ]  outPortNames=[' ']  dspbaimage=dspba_prim.jpg  text=fprintf('&');  style=Optimised  visibilities=8+2  version=20090407
  Const1 : DSPBAPrim/Const  primtype=const  nInputs=0  nOutputs=1  omode=Inherit via internal rule  otype=uint(8)  scale=1  rndmethod=Unbiased  factor=1  satmethod=Symmetric  shift_vec=[0 1 2 -1]  value=1  inPortNames=['+'; '+';]  outPortNames=[' ']  dspbaimage=dspba_prim.jpg  text=fprintf('%s', num2str(value));  style=Optimised  visibilities=8 + 1024  floatPrecision=float32_m23  version=20120820
  Const2 : DSPBAPrim/Const  primtype=const  nInputs=0  nOutputs=1  omode=Inherit via internal rule  otype=uint(8)  scale=1  rndmethod=Unbiased  factor=1  satmethod=Symmetric  shift_vec=[0 1 2 -1]  value=size  inPortNames=['+'; '+';]  outPortNames=[' ']  dspbaimage=dspba_prim.jpg  text=fprintf('%s', num2str(value));  style=Optimised  visibilities=8 + 1024  floatPrecision=float32_m23  version=20120820
  Const3 : DSPBAPrim/Const  primtype=const  nInputs=0  nOutputs=1  omode=Inherit via internal rule  otype=uint(nextpow2(row*row))  scale=1  rndmethod=Unbiased  factor=1  satmethod=Symmetric  shift_vec=[0 1 2 -1]  value=1  inPortNames=['+'; '+';]  outPortNames=[' ']  dspbaimage=dspba_prim.jpg  text=fprintf('%s', num2str(value));  style=Optimised  visibilities=8 + 1024  floatPrecision=float32_m23  version=20120820
  Const4 : DSPBAPrim/Const  primtype=const  nInputs=0  nOutputs=1  omode=Inherit via internal rule  otype=uint(nextpow2(row_count_1*column_count_2))  scale=1  rndmethod=Unbiased  factor=1  satmethod=Symmetric  shift_vec=[0 1 2 -1]  value=0  inPortNames=['+'; '+';]  outPortNames=[' ']  dspbaimage=dspba_prim.jpg  text=fprintf('%s', num2str(value));  style=Optimised  visibilities=8 + 1024  floatPrecision=float32_m23  version=20120820
  Const8 : DSPBAPrim/Const  primtype=const  nInputs=0  nOutputs=1  omode=Inherit via internal rule  otype=uint(8)  scale=1  rndmethod=Unbiased  factor=1  satmethod=Symmetric  shift_vec=[0 1 2 -1]  value=0  inPortNames=['+'; '+';]  outPortNames=[' ']  dspbaimage=dspba_prim.jpg  text=fprintf('%s', num2str(value));  style=Optimised  visibilities=8 + 1024  floatPrecision=float32_m23  version=20120820
  Delay : DSPBAPrim/SampleDelay  primtype=sampdelay  nInputs=1  nOutputs=1  omode=Inherit via internal rule  otype=sfix(16)  scale=2^-15  rndmethod=Unbiased  factor=1  satmethod=Symmetric  shift_vec=[0 1 2 -1]  value=1  inPortNames=[' '; ' ';]  outPortNames=[' ']  dspbaimage=dspba_prim.jpg  text=dpoly(1, eye(1,value+1), 'z')  style=Optimised  visibilities=8 + 1024 + 2^17 + 2^18  flexible=off  slackgroup=0  augmented=0  version=20090407  advOptions=[]
  LoadableCounter : DSPBAPrim/LoadableCounter  primtype=loadablecounter  nInputs=5  nOutputs=1  omode=Specify via dialog  otype=uint(nextpow2(size))  scale=1  rndmethod=Unbiased  factor=1  satmethod=Symmetric  shift_vec=[0 1 2 -1]  value=[0 (size) 1]  inPortNames=['en';'ld';'i ';'s ';'m ']  outPortNames=[' ']  dspbaimage=dspba_prim.jpg  text=fprintf('loadable\ncounter\n[%d %d %d]', value(1), value(2), value(3));  style=Optimised  visibilities=8 + 1024  version=20090407
  Output Read Logic : DSPBAPrim/ForLoop  looptest=<
  Read Delay : DSPBAPrim/SampleDelay  primtype=sampdelay  nInputs=1  nOutputs=1  omode=Inherit via internal rule  otype=sfix(16)  scale=2^-15  rndmethod=Unbiased  factor=1  satmethod=Symmetric  shift_vec=[0 1 2 -1]  value=2  inPortNames=[' '; ' ';]  outPortNames=[' ']  dspbaimage=dspba_prim.jpg  text=dpoly(1, eye(1,value+1), 'z')  style=Optimised  visibilities=8 + 1024 + 2^17 + 2^18  flexible=off  slackgroup=0  augmented=0  version=20090407  advOptions=[]
  Read Delay1 : DSPBAPrim/SampleDelay  primtype=sampdelay  nInputs=1  nOutputs=1  omode=Inherit via internal rule  otype=sfix(16)  scale=2^-15  rndmethod=Unbiased  factor=1  satmethod=Symmetric  shift_vec=[0 1 2 -1]  value=2  inPortNames=[' '; ' ';]  outPortNames=[' ']  dspbaimage=dspba_prim.jpg  text=dpoly(1, eye(1,value+1), 'z')  style=Optimised  visibilities=8 + 1024 + 2^17 + 2^18  flexible=off  slackgroup=0  augmented=0  version=20090407  advOptions=[]
  Read Delay2 : DSPBAPrim/SampleDelay  primtype=sampdelay  nInputs=1  nOutputs=1  omode=Inherit via internal rule  otype=sfix(16)  scale=2^-15  rndmethod=Unbiased  factor=1  satmethod=Symmetric  shift_vec=[0 1 2 -1]  value=2  inPortNames=[' '; ' ';]  outPortNames=[' ']  dspbaimage=dspba_prim.jpg  text=dpoly(1, eye(1,value+1), 'z')  style=Optimised  visibilities=8 + 1024 + 2^17 + 2^18  flexible=off  slackgroup=0  augmented=0  version=20090407  advOptions=[]
  ReinterpretCast_Result : DSPBAPrim/ReinterpretCast  primtype=reinterpret  nInputs=1  nOutputs=1  omode=Specify via dialog  otype=uint(nextpow2(size))  scale=1  rndmethod=Unbiased  factor=1  satmethod=Symmetric  shift_vec=[0 1 2 -1]  value=0  inPortNames=[' '; ' ';]  outPortNames=[' ']  dspbaimage=dspba_prim.jpg  text=fprintf('Reinterp\nCast', value);  style=Optimised  visibilities=8  floatPrecision=float32_m23  version=20120601
  Result RAM : DSPBAPrim/DualMem  primtype=dualmem  nInputs=4  nOutputs=2  omode=Inherit via internal rule  otype=sfix(16)  scale=2^-15  rndmethod=Unbiased  factor=1  satmethod=Symmetric  shift_vec=[0 1 2 -1]  value=zeros(size,1)  inPortNames=['d1'; 'a1'; 'w1'; 'a2']  outPortNames=['q1'; 'q2']  dspbaimage=dspba_prim.jpg  text=fprintf('dmem%s',AdvDSPBDMemDisplay(UseDontCare));  style=Optimised  visibilities=8 + 1024 + 2^17 + 2^18  UseDontCare=on  TwinWritePorts=off  version=20141001
  Rising Edge Detect : qrd_matrix_library/matrix_multiplication/Rising Edge Detect
  SRlatch : DSPBAControl/SRlatch
  Source Valid : Outport
  Source Data : Outport  Port=2
  Source SOP : Outport  Port=3
  Source EOP : Outport  Port=4
  Output_Busy : Outport  Port=5
  wires:
  Write Data/1 -> Result RAM/1
  Result RAM/2 -> Source Data/1
  Write Enable/1 -> Result RAM/3, LoadableCounter/1
  LoadableCounter/1 -> Result RAM/2
  Wr_Addr_Clr/1 -> LoadableCounter/2
  Const8/1 -> LoadableCounter/3
  Const1/1 -> LoadableCounter/4
  Const2/1 -> LoadableCounter/5
  Read Delay1/1 -> Source SOP/1
  Read Delay/1 -> Source Valid/1
  Source Ready/1 -> Output Read Logic/6, And/2
  Read Delay2/1 -> [Source_EOP], Source EOP/1
  Rising Edge Detect/1 -> Delay/1
  SRlatch/1 -> Output_Busy/1, And/1
  And/1 -> Rising Edge Detect/1
  Delay/1 -> Output Read Logic/2
  Output Read Logic/6 -> Read Delay/1
  Output Read Logic/7 -> ReinterpretCast_Result/1
  Output Read Logic/4 -> Read Delay1/1
  Output Read Logic/5 -> Read Delay2/1
  Const3/1 -> Output Read Logic/4
  Const4/1 -> Output Read Logic/3
  Output Read Logic/1 -> Output Read Logic/1
  [Source_EOP] -> SRlatch/2
  ReinterpretCast_Result/1 -> [Result_Read_Address]
  Done/1 -> SRlatch/1
  [Result_Read_Address] -> Result RAM/4
  Size/1 -> Output Read Logic/5

== system qrd_matrix_library/QR_decomposition/Q Output Memory Controller ==
  Write Enable : Inport
  Write Data : Inport  Port=2
  Wr_Addr_Clr : Inport  Port=3
  Done : Inport  Port=4
  Source Ready : Inport  Port=5
  Size : Inport  Port=6
  And : DSPBAPrim/And  primtype=and  nInputs=2  nOutputs=1  omode=Inherit via internal rule  otype=sfix(16)  scale=2^-15  rndmethod=Unbiased  factor=1  satmethod=Symmetric  shift_vec=[0 1 2 -1]  value=0  inPortNames=[' '; ' '; ' '; ' '; ' '; ' '; ' '; ' '; ' '; ' '; ' '; ' '; ' '; ' '; ' '; ' '; ]  outPortNames=[' ']  dspbaimage=dspba_prim.jpg  text=fprintf('&');  style=Optimised  visibilities=8+2  version=20090407
  Const1 : DSPBAPrim/Const  primtype=const  nInputs=0  nOutputs=1  omode=Inherit via internal rule  otype=uint(8)  scale=1  rndmethod=Unbiased  factor=1  satmethod=Symmetric  shift_vec=[0 1 2 -1]  value=1  inPortNames=['+'; '+';]  outPortNames=[' ']  dspbaimage=dspba_prim.jpg  text=fprintf('%s', num2str(value));  style=Optimised  visibilities=8 + 1024  floatPrecision=float32_m23  version=20120820
  Const2 : DSPBAPrim/Const  primtype=const  nInputs=0  nOutputs=1  omode=Inherit via internal rule  otype=uint(8)  scale=1  rndmethod=Unbiased  factor=1  satmethod=Symmetric  shift_vec=[0 1 2 -1]  value=size*size/vectorization  inPortNames=['+'; '+';]  outPortNames=[' ']  dspbaimage=dspba_prim.jpg  text=fprintf('%s', num2str(value));  style=Optimised  visibilities=8 + 1024  floatPrecision=float32_m23  version=20120820
  Const3 : DSPBAPrim/Const  primtype=const  nInputs=0  nOutputs=1  omode=Inherit via internal rule  otype=uint(nextpow2(row*row))  scale=1  rndmethod=Unbiased  factor=1  satmethod=Symmetric  shift_vec=[0 1 2 -1]  value=1  inPortNames=['+'; '+';]  outPortNames=[' ']  dspbaimage=dspba_prim.jpg  text=fprintf('%s', num2str(value));  style=Optimised  visibilities=8 + 1024  floatPrecision=float32_m23  version=20120820
  Const4 : DSPBAPrim/Const  primtype=const  nInputs=0  nOutputs=1  omode=Inherit via internal rule  otype=uint(nextpow2(row_count_1*column_count_2))  scale=1  rndmethod=Unbiased  factor=1  satmethod=Symmetric  shift_vec=[0 1 2 -1]  value=0  inPortNames=['+'; '+';]  outPortNames=[' ']  dspbaimage=dspba_prim.jpg  text=fprintf('%s', num2str(value));  style=Optimised  visibilities=8 + 1024  floatPrecision=float32_m23  version=20120820
  Const5 : DSPBAPrim/Const  primtype=const  nInputs=0  nOutputs=1  omode=Inherit via internal rule  otype=uint(8)  scale=1  rndmethod=Unbiased  factor=1  satmethod=Symmetric  shift_vec=[0 1 2 -1]  value=nextpow2(vectorization)  inPortNames=['+'; '+';]  outPortNames=[' ']  dspbaimage=dspba_prim.jpg  text=fprintf('%s', num2str(value));  style=Optimised  visibilities=8 + 1024  floatPrecision=float32_m23  version=20120820
  Const8 : DSPBAPrim/Const  primtype=const  nInputs=0  nOutputs=1  omode=Inherit via internal rule  otype=uint(8)  scale=1  rndmethod=Unbiased  factor=1  satmethod=Symmetric  shift_vec=[0 1 2 -1]  value=0  inPortNames=['+'; '+';]  outPortNames=[' ']  dspbaimage=dspba_prim.jpg  text=fprintf('%s', num2str(value));  style=Optimised  visibilities=8 + 1024  floatPrecision=float32_m23  version=20120820
  Delay : DSPBAPrim/SampleDelay  primtype=sampdelay  nInputs=1  nOutputs=1  omode=Inherit via internal rule  otype=sfix(16)  scale=2^-15  rndmethod=Unbiased  factor=1  satmethod=Symmetric  shift_vec=[0 1 2 -1]  value=1  inPortNames=[' '; ' ';]  outPortNames=[' ']  dspbaimage=dspba_prim.jpg  text=dpoly(1, eye(1,value+1), 'z')  style=Optimised  visibilities=8 + 1024 + 2^17 + 2^18  flexible=off  slackgroup=0  augmented=0  version=20090407  advOptions=[]
  LoadableCounter : DSPBAPrim/LoadableCounter  primtype=loadablecounter  nInputs=5  nOutputs=1  omode=Specify via dialog  otype=uint(nextpow2(size*size/vectorization))  scale=1  rndmethod=Unbiased  factor=1  satmethod=Symmetric  shift_vec=[0 1 2 -1]  value=[0 (size*size) 1]  inPortNames=['en';'ld';'i ';'s ';'m ']  outPortNames=[' ']  dspbaimage=dspba_prim.jpg  text=fprintf('loadable\ncounter\n[%d %d %d]', value(1), value(2), value(3));  style=Optimised  visibilities=8 + 1024  version=20090407
  Mult : DSPBAPrim/Mult  primtype=mult  nInputs=2  nOutputs=1  omode=Inherit via internal rule  otype=sfix(16)  scale=2^-15  rndmethod=Unbiased  factor=1  satmethod=Symmetric  shift_vec=[0 1 2 -1]  value=0  inPortNames=[' '; ' ';]  outPortNames=[' ']  dspbaimage=dspba_prim.jpg  text=fprintf('X');  style=Optimised  visibilities=8+2^18+2^19  floatPrecision=float32_m23  floatRounding=correct  advOptions=[]  version=20130115
  Output Read Logic : DSPBAPrim/ForLoop  looptest=<
  Read Delay : DSPBAPrim/SampleDelay  primtype=sampdelay  nInputs=1  nOutputs=1  omode=Inherit via internal rule  otype=sfix(16)  scale=2^-15  rndmethod=Unbiased  factor=1  satmethod=Symmetric  shift_vec=[0 1 2 -1]  value=2  inPortNames=[' '; ' ';]  outPortNames=[' ']  dspbaimage=dspba_prim.jpg  text=dpoly(1, eye(1,value+1), 'z')  style=Optimised  visibilities=8 + 1024 + 2^17 + 2^18  flexible=off  slackgroup=0  augmented=0  version=20090407  advOptions=[]
  Read Delay1 : DSPBAPrim/SampleDelay  primtype=sampdelay  nInputs=1  nOutputs=1  omode=Inherit via internal rule  otype=sfix(16)  scale=2^-15  rndmethod=Unbiased  factor=1  satmethod=Symmetric  shift_vec=[0 1 2 -1]  value=2  inPortNames=[' '; ' ';]  outPortNames=[' ']  dspbaimage=dspba_prim.jpg  text=dpoly(1, eye(1,value+1), 'z')  style=Optimised  visibilities=8 + 1024 + 2^17 + 2^18  flexible=off  slackgroup=0  augmented=0  version=20090407  advOptions=[]
  Read Delay2 : DSPBAPrim/SampleDelay  primtype=sampdelay  nInputs=1  nOutputs=1  omode=Inherit via internal rule  otype=sfix(16)  scale=2^-15  rndmethod=Unbiased  factor=1  satmethod=Symmetric  shift_vec=[0 1 2 -1]  value=2  inPortNames=[' '; ' ';]  outPortNames=[' ']  dspbaimage=dspba_prim.jpg  text=dpoly(1, eye(1,value+1), 'z')  style=Optimised  visibilities=8 + 1024 + 2^17 + 2^18  flexible=off  slackgroup=0  augmented=0  version=20090407  advOptions=[]
  ReinterpretCast_Result : DSPBAPrim/ReinterpretCast  primtype=reinterpret  nInputs=1  nOutputs=1  omode=Specify via dialog  otype=uint(nextpow2(size*size))  scale=1  rndmethod=Unbiased  factor=1  satmethod=Symmetric  shift_vec=[0 1 2 -1]  value=0  inPortNames=[' '; ' ';]  outPortNames=[' ']  dspbaimage=dspba_prim.jpg  text=fprintf('Reinterp\nCast', value);  style=Optimised  visibilities=8  floatPrecision=float32_m23  version=20120601
  Result RAM : DSPBAPrim/DualMem  primtype=dualmem  nInputs=4  nOutputs=2  omode=Inherit via internal rule  otype=sfix(16)  scale=2^-15  rndmethod=Unbiased  factor=1  satmethod=Symmetric  shift_vec=[0 1 2 -1]  value=complex(zeros(size*size,1),zeros(size*size,1))  inPortNames=['d1'; 'a1'; 'w1'; 'a2']  outPortNames=['q1'; 'q2']  dspbaimage=dspba_prim.jpg  text=fprintf('dmem%s',AdvDSPBDMemDisplay(UseDontCare));  style=Optimised  visibilities=8 + 1024 + 2^17 + 2^18  UseDontCare=on  TwinWritePorts=off  version=20141001
  Rising Edge Detect : qrd_matrix_library/matrix_multiplication/Rising Edge Detect
  SRlatch : DSPBAControl/SRlatch
  Shift : DSPBAPrim/Shift  primtype=shift  nInputs=2  nOutputs=1  omode=Inherit via internal rule  otype=sfix(16)  scale=2^-15  rndmethod=Unbiased  factor=1  satmethod=Symmetric  shift_vec=[0 1 2 -1]  value=0  inPortNames=['a'; 'b';]  outPortNames=[' ']  dspbaimage=dspba_prim.jpg  text=fprintf('a >> b');  style=Optimised  visibilities=8  version=20090407
  Source Valid : Outport
  Source Data : Outport  Port=2
  Source SOP : Outport  Port=3
  Source EOP : Outport  Port=4
  Output_Busy : Outport  Port=5
  wires:
  Write Data/1 -> Result RAM/1
  Result RAM/2 -> Source Data/1
  Write Enable/1 -> Result RAM/3, LoadableCounter/1
  LoadableCounter/1 -> Result RAM/2
  Wr_Addr_Clr/1 -> LoadableCounter/2
  Const8/1 -> LoadableCounter/3
  Const1/1 -> LoadableCounter/4
  Const2/1 -> LoadableCounter/5
  Read Delay1/1 -> Source SOP/1
  Read Delay/1 -> Source Valid/1
  Source Ready/1 -> Output Read Logic/6, And/2
  Read Delay2/1 -> [Source_EOP], Source EOP/1
  Rising Edge Detect/1 -> Delay/1
  SRlatch/1 -> Output_Busy/1, And/1
  And/1 -> Rising Edge Detect/1
  Delay/1 -> Output Read Logic/2
  Output Read Logic/6 -> Read Delay/1
  Output Read Logic/7 -> ReinterpretCast_Result/1
  Output Read Logic/4 -> Read Delay1/1
  Output Read Logic/5 -> Read Delay2/1
  Mult/1 -> Shift/1
  Const3/1 -> Output Read Logic/4
  Const4/1 -> Output Read Logic/3
  Output Read Logic/1 -> Output Read Logic/1
  [Source_EOP] -> SRlatch/2
  Size/1 -> Mult/2, Mult/1
  ReinterpretCast_Result/1 -> [Result_Read_Address]
  Done/1 -> SRlatch/1
  [Result_Read_Address] -> Result RAM/4
  Shift/1 -> Output Read Logic/5
  Const5/1 -> Shift/2
